simulink model "OS4dynamics_01"  (R2017b)
settings: Solver=ode45  StartTime=0.0  StopTime=10  RelTol=1e-3  EnableMultiTasking=on
InitFcn:
  | OS4dynamics_01_init
undefined symbols (not defined in the file or in its folder): Newton, OS4_initC, OS4_initR, OS4_initX, OS4_physical, Raphson
libraries: QuaternionLib x12, simulink x2
settings Model: Creator=EwingKang  LastModifiedBy=KingBoy
settings SolverCC: ZeroCrossAlgorithm=Adaptive
settings DataIOCC: LimitDataPoints=on  SaveFormat=Array  SaveOutput=off  SaveTime=off
settings OptimizationCC: DefaultParameterBehavior=Inlined  LifeSpan=inf
settings DebuggingCC: SolverPrmCheckMsg=warning  StateNameClashWarn=warning  StrictBusMsg=ErrorOnBusTreatedAsVector  SFUnexpectedBacktrackingDiag=warning  SFNoUnconditionalDefaultTransitionDiag=warning  SFExecutionAtInitializationDiag=none
settings HardwareCC: ProdBitPerPointer=32  ProdBitPerSizeT=32  ProdBitPerPtrDiffT=32  ProdLargestAtomicFloat=None  ProdIntDivRoundTo=Undefined  ProdEndianess=Unspecified  ProdWordSize=32  ProdHWDeviceType=32-bit Generic
settings ModelReferenceCC: ModelReferenceNumInstancesAllowed=Single  ModelReferencePassRootInputsByReference=off  PropagateSignalLabelsOutOfModel=off
settings CodeAppCC: StateflowObjectComments=on
settings GRTTargetCC: TargetLangStandard=C89/C90 (ANSI)  GeneratePreprocessorConditionals=Disable all
settings ConfigComp: CovMetricSettings=dw  CovHtmlReporting=on  CovSaveCumulativeToWorkspaceVar=on  CovSaveSingleToWorkspaceVar=on  CovExternalEMLEnable=off  CovSFcnEnable=off
settings SimscapeCC: EditingMode=Restricted  SimscapeNormalizeSystem=off
settings ConfigurationSet: Description=SimMechanics 2G

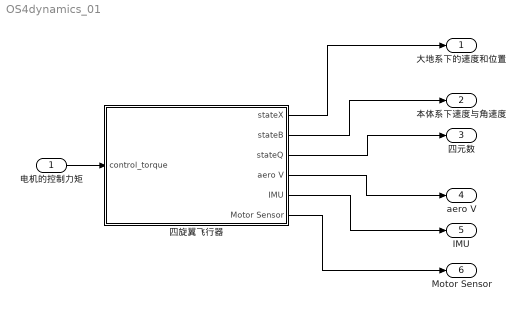
== system OS4dynamics_01 ==
  电机的控制力矩 : Inport  PortDimensions=4
  四旋翼飞行器 : Subsystem
  大地系下的速度和位置 : Outport
  本体系下速度与角速度 : Outport  Port=2
  四元数 : Outport  Port=3
  aero V : Outport  Port=4
  IMU : Outport  Port=5
  Motor Sensor : Outport  Port=6
  wires:
  电机的控制力矩/1 -> 四旋翼飞行器/1(control_torque)
  四旋翼飞行器/1(stateX) -> 大地系下的速度和位置/1
  四旋翼飞行器/2(stateB) -> 本体系下速度与角速度/1
  四旋翼飞行器/3(stateQ) -> 四元数/1
  四旋翼飞行器/4(aero V) -> aero V/1
  四旋翼飞行器/5(IMU) -> IMU/1
  四旋翼飞行器/6(Motor Sensor) -> Motor Sensor/1

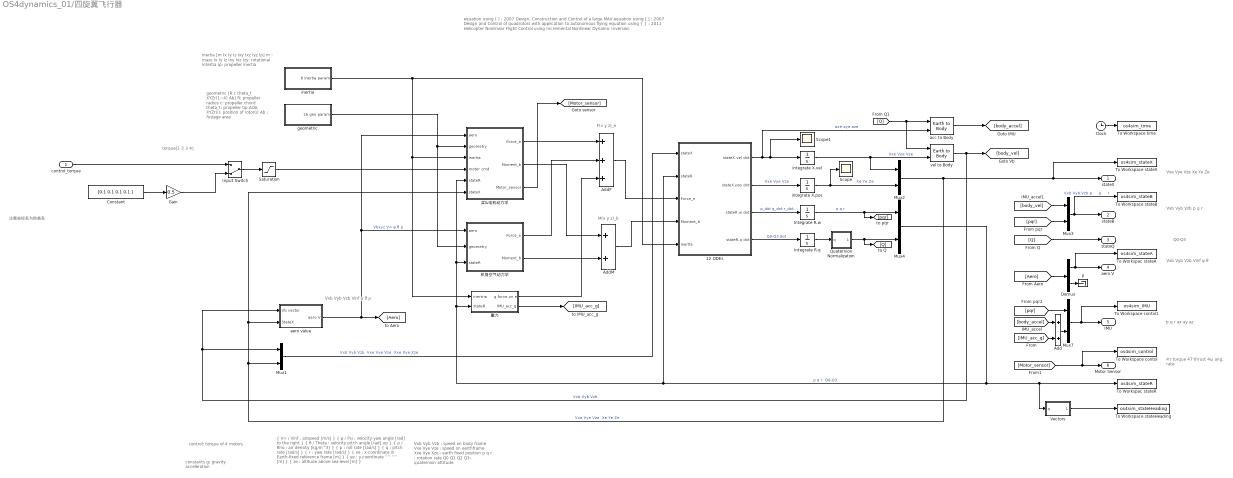
== system OS4dynamics_01/四旋翼飞行器 ==
  note: 注意坐标系为欧美系
  note: equation using ( ) : 2007 Design, Construction and Control of a large MAV
      | equation using [ ] : 2007 Design and Control of quadrotors with application to autonomous flying
      | equation using { } : 2011 Helicopter Nonlinear Flight Control using Incremental Nonlinear Dynamic Inversion
  note: Q0-Q3
  note: constants
      | g: gravity acceleration
  note: control:
      |   torque of 4 motors
  note: Vxb  Vyb Vzb : speed on body frame
      | Vxe Vye Vze  : speed on earthframe
      | Xxe Xye Xze  : earth fixed position
      | p q r               : rotation rate
      | Q0 Q1 Q2 Q3: quaternion attitude
  note: Vxb Vyb Vzb
      | p     q     r
  note: Vxe Vye Vze
      | Xe   Ye   Ze
  note: { V∞ / Vinf : airspeed [m/s] }
      | { ψ / Psi : velocity yaw angle [rad] to the right }
      | { θ / Theta : velocity pitch angle [rad] up }
      | { ρ / Rho : air density [kg/m^3] }
      | { p : roll rate [rad/s] }
      | { q : pitch rate [rad/s] }
      | { r : yaw rate [rad/s] }
      | { xe : x-coordinate in Earth-fixed reference frame [m] }
      | { ye : y-coordinate '' '' '' '' [m] }
      | { ze : altitude above sea-level [m] }
  note: torque[1 2 3 4]
  note: M(x y z)_b
  note: F(x y z)_e
  note: p q r ax ay az
  note: inertia
      | [m Ix Iy Iz Ixy Ixz Iyz Ip]
      | m : mass
      | Ix Iy Iz Ixy Ixz Izy: rotational intertia
      | Ip: propeller inertia
  note: geometric
      |  [R c theta_t XYZr(1~4) Ab]
      |
      | R:         propeller radius
      | c:          propeller chord
      | theta_t: propeller tip AOA
      | XYZr(i): position of rotor(i)
      | Ab      : fuslage area
  note: Vxb Vyb Vzb
      | Vinf ψ θ ρ
  note: Vxb Vyb Vzb
      | Vinf ψ θ
  note: 4τ torque
      | 4T thrust
      | 4ω ang. rate
  control_torque : Inport  PortDimensions=4
  12 ODEs : Subsystem
  Add : Sum
  AddF : Sum  Inputs=+++
  AddM : Sum
  Clock : Clock
  Constant : Constant  Value=[0.1 0.1 0.1 0.1 ]
  Demux : Demux  Outputs=[6 1 ]
  Gain : Gain  Gain=0.5
  Input Switch : ManualSwitch  CurrentSetting=0
  Integrate R.q : Integrator  InitialCondition=OS4_initR.q
  Integrate R.w : Integrator  InitialCondition=OS4_initR.w
  Mux{1..4,7} (5 alike) : Mux  Inputs=2
  Quaternion Normalization : Subsystem
  Saturation : Saturate  UpperLimit=0.2  LowerLimit=0
  Scope : Scope
  Scope1 : Scope
  To Workspac stateA : ToWorkspace  VariableName=os4sim_stateA  SaveFormat=Timeseries  SampleTime=-1
  To Workspac stateR : ToWorkspace  VariableName=os4sim_stateR  SaveFormat=Timeseries  SampleTime=-1
  To Workspace contol : ToWorkspace  VariableName=os4sim_control  SaveFormat=Timeseries  SampleTime=-1
  To Workspace contol1 : ToWorkspace  VariableName=os4sim_IMU  SaveFormat=Timeseries  SampleTime=-1
  To Workspace stateB : ToWorkspace  VariableName=os4sim_stateB  SaveFormat=Timeseries  SampleTime=-1
  To Workspace stateHeading : ToWorkspace  VariableName=os4sim_stateHeading  SaveFormat=Timeseries  SampleTime=-1
  To Workspace stateX : ToWorkspace  VariableName=os4sim_stateX  SaveFormat=Timeseries  SampleTime=-1
  To Workspace time : ToWorkspace  VariableName=os4sim_time  SaveFormat=Timeseries  SampleTime=-1
  Vectors : Subsystem
  acc to Body : QuaternionLib/Earth to Body
  aero value : Subsystem
  geometric : Subsystem
  inertia : Subsystem
  integrate X.pos : Integrator  InitialCondition=OS4_initX.pos
  integrate X.vel : Integrator  InitialCondition=OS4_initX.vel
  vel to Body : QuaternionLib/Earth to Body
  ρ : Terminator
  机身空气动力学 : Subsystem
  桨&电机动力学 : Subsystem
  重力 : Subsystem
  stateX : Outport
  stateB : Outport  Port=2
  stateQ : Outport  Port=3
  aero V : Outport  Port=4
  IMU : Outport  Port=5
  Motor Sensor : Outport  Port=6
  wires:
  Mux2/1 -> stateX/1, To Workspace stateX/1, 桨&电机动力学/6(stateX), aero value/2(StateX), Mux1/2  "Vxe Vye Vze  Xe Ye Ze"
  Mux1/1 -> 12 ODEs/1(stateX)  "Vxb Vyb Vzb  Vxe Vye Vze  Xxe Xye Xze"
  桨&电机动力学/1(Force_e) -> AddF/1
  Mux4/1 -> Vectors/1(q), To Workspac stateR/1, 12 ODEs/2(stateR), 重力/2(stateR), 桨&电机动力学/5(stateR), 机身空气动力学/3(stateR)  "p q r  Q0-Q3"
  12 ODEs/1(stateX.vel dot) -> acc to Body/2, Scope1/1, integrate X.vel/1  "axe aye aze"
  12 ODEs/3("stateR.w dot ") -> Integrate R.w/1  "p_dot q_dot r_dot"
  geometric/1(16 geo param) -> 机身空气动力学/2(geometry), 桨&电机动力学/2(geometry)
  aero value/1(aero V) -> [Aero], 桨&电机动力学/1(aero), 机身空气动力学/1(aero)  "Vbxyz V∞ ψ θ ρ"
  AddF/1 -> 12 ODEs/3(Force_e)
  重力/1(g force on e) -> AddF/3
  Clock/1 -> To Workspace time/1
  Quaternion Normalization/1(qnorm) -> Mux4/2, [Q]
  integrate X.vel/1 -> vel to Body/2, Mux2/1  "Vxe Vye Vze"
  vel to Body/1 -> [body_vel], aero value/1(Vb vector), Mux1/1  "Vxb Vyb Vzb"
  AddM/1 -> 12 ODEs/4(Moment_b)
  [body_accel] -> Add/1
  [Q] -> vel to Body/1, acc to Body/1
  Saturation/1 -> 桨&电机动力学/4(motor cmd)
  12 ODEs/4(stateR.q dot) -> Integrate R.q/1  "Q0-Q3 dot"
  Mux3/1 -> stateB/1, To Workspace stateB/1  "Vxb Vyb Vzb p     q     r"
  桨&电机动力学/2(Moment_b) -> AddM/1
  [Aero] -> Demux/1
  [Motor_sensor] -> Motor Sensor/1, To Workspace contol/1
  Demux/2 -> ρ/1
  control_torque/1 -> Input Switch/1
  [body_vel] -> Mux3/1
  桨&电机动力学/3(Motor_sensor) -> [Motor_sensor]
  12 ODEs/2(stateX.pos dot) -> integrate X.pos/1  "Vxe Vye Vze"
  重力/2(IMU_acc_g) -> [IMU_acc_g]
  Mux7/1 -> IMU/1, To Workspace contol1/1
  Demux/1 -> aero V/1, To Workspac stateA/1
  Integrate R.q/1 -> Quaternion Normalization/1(q)
  机身空气动力学/1(Force_e) -> AddF/2
  Add/1 -> Mux7/2
  integrate X.pos/1 -> Scope/1, Mux2/2  "Xe Ye Ze"
  Vectors/1(Vector) -> To Workspace stateHeading/1
  [Q] -> stateQ/1
  [pqr] -> Mux7/1
  [IMU_acc_g] -> Add/2
  机身空气动力学/2(Moment_b) -> AddM/2
  Integrate R.w/1 -> Mux4/1, [pqr]  "p q r"
  acc to Body/1 -> [body_accel]
  [pqr] -> Mux3/2
  Input Switch/1 -> Saturation/1
  inertia/1(8 inertia param) -> 12 ODEs/5(Inertia), 桨&电机动力学/3(inertia), 重力/1(inertria)
  Constant/1 -> Gain/1
  Gain/1 -> Input Switch/2

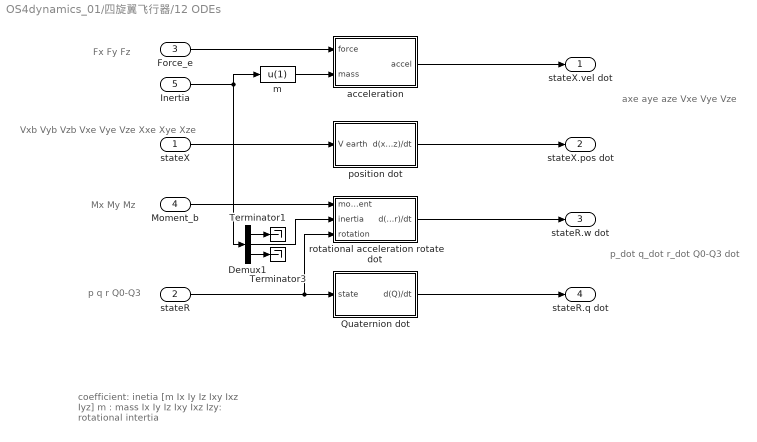
== system OS4dynamics_01/四旋翼飞行器/12 ODEs ==
  note: p_dot q_dot r_dot
      | Q0-Q3 dot
  note: axe aye aze
      | Vxe Vye Vze
  note: Vxb Vyb Vzb Vxe Vye Vze Xxe Xye Xze
  note: Mx My Mz
  note: Fx Fy Fz
  note: p q r Q0-Q3
  note: coefficient: inetia
      | [m Ix Iy Iz Ixy Ixz Iyz]
      | m : mass
      | Ix Iy Iz Ixy Ixz Izy: rotational intertia
  stateX : Inport
  stateR : Inport  Port=2
  Force_e : Inport  Port=3
  Moment_b : Inport  Port=4
  Inertia : Inport  Port=5
  Demux1 : Demux  Outputs=[1 3 4]
  Quaternion dot : Subsystem
  Terminator1 : Terminator
  Terminator3 : Terminator
  acceleration : Subsystem
  m : Fcn  Expr=u(1)
  position dot : Subsystem
  rotational acceleration rotate dot : Subsystem
  stateX.vel dot : Outport
  stateX.pos dot : Outport  Port=2
  "stateR.w dot " : Outport  Port=3
  stateR.q dot : Outport  Port=4
  wires:
  Inertia/1 -> m/1, Demux1/1
  Moment_b/1 -> rotational acceleration rotate dot/1(moment)
  Force_e/1 -> acceleration/1(force)
  stateR/1 -> rotational acceleration rotate dot/3(rotation), Quaternion dot/1(state)
  acceleration/1(accel) -> stateX.vel dot/1
  position dot/1(d(xyz)/dt) -> stateX.pos dot/1
  rotational acceleration rotate dot/1(d(pqr)/dt) -> "stateR.w dot "/1
  stateX/1 -> position dot/1(V earth)
  m/1 -> acceleration/2(mass)
  Demux1/2 -> rotational acceleration rotate dot/2(inertia)
  Demux1/1 -> Terminator1/1
  Demux1/3 -> Terminator3/1
  Quaternion dot/1(d(Q)/dt) -> stateR.q dot/1

== system OS4dynamics_01/四旋翼飞行器/Quaternion Normalization ==
  q : Inport  PortDimensions=4
  Product : Product  Inputs=*/  SaturateOnIntegerOverflow=on  RndMeth=Zero  InputSameDT=on  OutDataTypeStr=Inherit: Same as first input
  Square : Math  Operator=square  SaturateOnIntegerOverflow=on
  Square Root : Sqrt  Operator=signedSqrt  AlgorithmType=Newton-Raphson  SaturateOnIntegerOverflow=on
  Sum : Sum  Inputs=1  SaturateOnIntegerOverflow=on  InputSameDT=on  OutDataTypeStr=Inherit: Same as first input
  qnorm : Outport  PortDimensions=4
  wires:
  Product/1 -> qnorm/1
  Square Root/1 -> Product/2
  Square/1 -> Sum/1
  Sum/1 -> Square Root/1
  q/1 -> Product/1, Square/1

== system OS4dynamics_01/四旋翼飞行器/Vectors ==
  q : Inport
  1,0,0 : Subsystem
  1,0,1 : Subsystem
  Body to Earth w/R1 : QuaternionLib/Body to Earth w//R
  Body to Earth w/R2 : QuaternionLib/Body to Earth w//R
  Mux6 : Mux  Inputs=2
  Vector : Outport
  wires:
  1,0,0/1(1,0,0) -> Body to Earth w/R1/2
  Body to Earth w/R1/1 -> Mux6/1
  q/1 -> Body to Earth w/R1/1, Body to Earth w/R2/1  "p q r  Q0-Q3"
  Mux6/1 -> Vector/1
  Body to Earth w/R2/1 -> Mux6/2
  1,0,1/1(0,1,0) -> Body to Earth w/R2/2

== system OS4dynamics_01/四旋翼飞行器/aero value ==
  note: Vxb Vyb Vzb
      | Vinf
      | ψ
      | θ
      | ρ
  note: Vxb Vyb Vzb
  Vb vector : Inport
  StateX : Inport  Port=2
  Compare To Constant : simulink/Logic and Bit Operations/Compare To Constant  relop=>  const=0  OutDataTypeStr=boolean
  Constant : Constant  Value=inf
  Mux : Mux  Inputs=5
  Mux1 : Mux  Inputs=2
  Switch : Switch  Criteria=u2 > Threshold
  Vinf alpha beta : Display
  Vinfinity : Fcn  Expr=sqrt(u(1)^2+u(2)^2+u(3)^2)
  Vx Vy Vz : Display
  altitude air density : Fcn  Expr=1.23
  θ asin ( -Vz / Vinf) : Fcn  Expr=asin(-u(4) / u(1))
  ψ atan( Vy / Vx ) : Fcn  Expr=atan2( u(2),u(1) )
  aero V : Outport
  wires:
  Switch/1 -> Mux/2, Mux1/1
  θ asin ( -Vz / Vinf)/1 -> Mux/4
  Mux/1 -> Vinf alpha beta/1, aero V/1
  ψ atan( Vy / Vx )/1 -> Mux/3
  Mux1/1 -> θ asin ( -Vz / Vinf)/1
  altitude air density/1 -> Mux/5
  StateX/1 -> altitude air density/1
  Vb vector/1 -> Vinfinity/1, ψ atan( Vy / Vx )/1, Mux1/2, Vx Vy Vz/1, Mux/1
  Vinfinity/1 -> Switch/1, Compare To Constant/1
  Compare To Constant/1 -> Switch/2
  Constant/1 -> Switch/3

== system OS4dynamics_01/四旋翼飞行器/geometric ==
  note: geometric
      |  [R c theta_t XYZr(1~4) Ab]
      |
      | R:         propeller radius
      | c:          propeller chord
      | theta_t: propeller tip AOA
      | XYZr(i): position of rotor(i)
      | Ab      : fuslage area
  Mux6 : Mux  Inputs=8
  Propeller Chord c : Constant  Value=OS4_physical.prop.chord
  Propeller tip AOA : Constant  Value=OS4_physical.prop.thetatip
  body area Ab : Constant  Value=OS4_physical.size.fuselage.area
  propeller Radius R : Constant  Value=OS4_physical.prop.rad
  rotor1 pos XYZr1 : Constant  Value=OS4_physical.rotor.pos(1:3,1)
  rotor1 pos XYZr2 : Constant  Value=OS4_physical.rotor.pos(1:3,2)
  rotor1 pos XYZr3 : Constant  Value=OS4_physical.rotor.pos(1:3,3)
  rotor1 pos XYZr4 : Constant  Value=OS4_physical.rotor.pos(1:3,4)
  16 geo param : Outport
  wires:
  Mux6/1 -> 16 geo param/1
  propeller Radius R/1 -> Mux6/1
  Propeller Chord c/1 -> Mux6/3
  rotor1 pos XYZr1/1 -> Mux6/4
  rotor1 pos XYZr2/1 -> Mux6/5
  rotor1 pos XYZr3/1 -> Mux6/6
  rotor1 pos XYZr4/1 -> Mux6/7
  body area Ab/1 -> Mux6/8
  Propeller tip AOA/1 -> Mux6/2

== system OS4dynamics_01/四旋翼飞行器/inertia ==
  note: inertia
      | [m Ix Iy Iz Ixy Ixz Iyz Ip]
      | m : mass
      | Ix Iy Iz Ixy Ixz Izy: rotational intertia
      | Ip: propeller inertia
  Ip : Constant  Value=OS4_physical.inertia.Ip
  Ix : Constant  Value=OS4_physical.inertia.Ixx
  Ixy : Constant  Value=OS4_physical.inertia.Ixy
  Ixz : Constant  Value=OS4_physical.inertia.Ixz
  Iy : Constant  Value=OS4_physical.inertia.Iyy
  Iyz : Constant  Value=OS4_physical.inertia.Iyz
  Iz : Constant  Value=OS4_physical.inertia.Izz
  Mux : Mux  Inputs=2
  Mux1 : Mux  Inputs=2
  Mux2 : Mux  Inputs=2
  Mux6 : Mux  Inputs=5
  m : Constant  Value=OS4_physical.inertia.mass
  8 inertia param : Outport
  wires:
  Ix/1 -> Mux/1
  Iy/1 -> Mux/2
  Ixz/1 -> Mux2/1
  Iyz/1 -> Mux2/2
  Iz/1 -> Mux1/1
  Ixy/1 -> Mux1/2
  Mux6/1 -> 8 inertia param/1
  m/1 -> Mux6/1
  Mux/1 -> Mux6/2
  Mux1/1 -> Mux6/3
  Mux2/1 -> Mux6/4
  Ip/1 -> Mux6/5

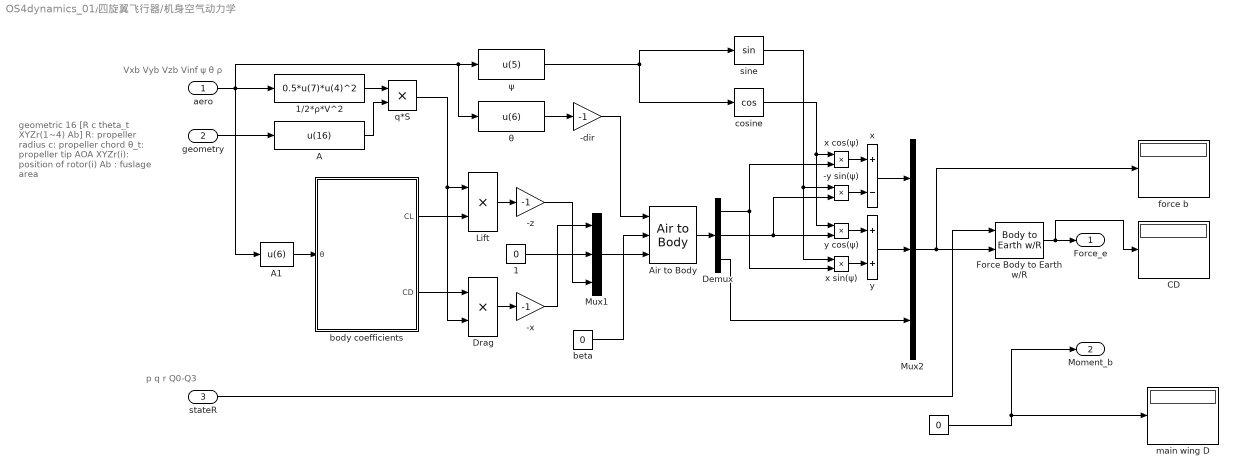
== system OS4dynamics_01/四旋翼飞行器/机身空气动力学 ==
  note: p q r
      | Q0-Q3
  note: Vxb Vyb Vzb
      | Vinf ψ θ ρ
  note: geometric 16
      | [R c theta_t XYZr(1~4) Ab]
      |
      | R: propeller radius
      | c: propeller chord
      | θ_t: propeller tip AOA
      | XYZr(i): position of rotor(i)
      | Ab : fuslage area
  aero : Inport  PortDimensions=7
  geometry : Inport  Port=2
  stateR : Inport  Port=3
  "  " : Constant  Value=0
  " 1" : Constant  Value=0
  -dir : Gain  Gain=-1
  -x : Gain  Gain=-1
  -y sin(ψ) : Product
  -z : Gain  Gain=-1
  1/2*ρ*V^2 : Fcn  Expr=0.5*u(7)*u(4)^2
  A : Fcn  Expr=u(16)
  A1 : Fcn  Expr=u(6)
  Air to Body : QuaternionLib/Air to Body
  CD : Display
  Demux : Demux  Outputs=3
  Drag : Product
  Force Body to Earth w/R : QuaternionLib/Body to Earth w//R
  Lift : Product
  Mux1 : Mux  Inputs=3
  Mux2 : Mux  Inputs=3
  beta : Constant  Value=0
  body coefficients : Subsystem
  cosine : Trigonometry  Operator=cos
  force b : Display
  main wing D : Display
  q*S : Product
  sine : Trigonometry
  x : Sum  Inputs=+-
  x cos(ψ) : Product
  x sin(ψ) : Product
  y : Sum
  y cos(ψ) : Product
  θ : Fcn  Expr=u(6)
  ψ : Fcn  Expr=u(5)
  Force_e : Outport
  Moment_b : Outport  Port=2
  wires:
  Force Body to Earth w/R/1 -> CD/1, Force_e/1
  stateR/1 -> Force Body to Earth w/R/1
  geometry/1 -> A/1
  1/2*ρ*V^2/1 -> q*S/1
  A/1 -> q*S/2
  q*S/1 -> Lift/1, Drag/2
  "  "/1 -> main wing D/1, Moment_b/1
  aero/1 -> A1/1, θ/1, ψ/1, 1/2*ρ*V^2/1
  body coefficients/2(CD) -> Drag/1
  body coefficients/1(CL) -> Lift/2
  A1/1 -> body coefficients/1(θ)
  Drag/1 -> -x/1
  -x/1 -> Mux1/1
  Lift/1 -> -z/1
  -z/1 -> Mux1/3
  " 1"/1 -> Mux1/2
  θ/1 -> -dir/1
  -dir/1 -> Air to Body/1
  Mux1/1 -> Air to Body/3
  beta/1 -> Air to Body/2
  Air to Body/1 -> Demux/1
  ψ/1 -> sine/1, cosine/1
  x/1 -> Mux2/1
  y/1 -> Mux2/2
  cosine/1 -> y cos(ψ)/1, x cos(ψ)/1
  Demux/1 -> x sin(ψ)/2, x cos(ψ)/2
  Demux/3 -> Mux2/3
  x sin(ψ)/1 -> y/2
  x cos(ψ)/1 -> x/1
  -y sin(ψ)/1 -> x/2
  y cos(ψ)/1 -> y/1
  Demux/2 -> -y sin(ψ)/2, y cos(ψ)/2
  sine/1 -> -y sin(ψ)/1, x sin(ψ)/1
  Mux2/1 -> force b/1, Force Body to Earth w/R/2

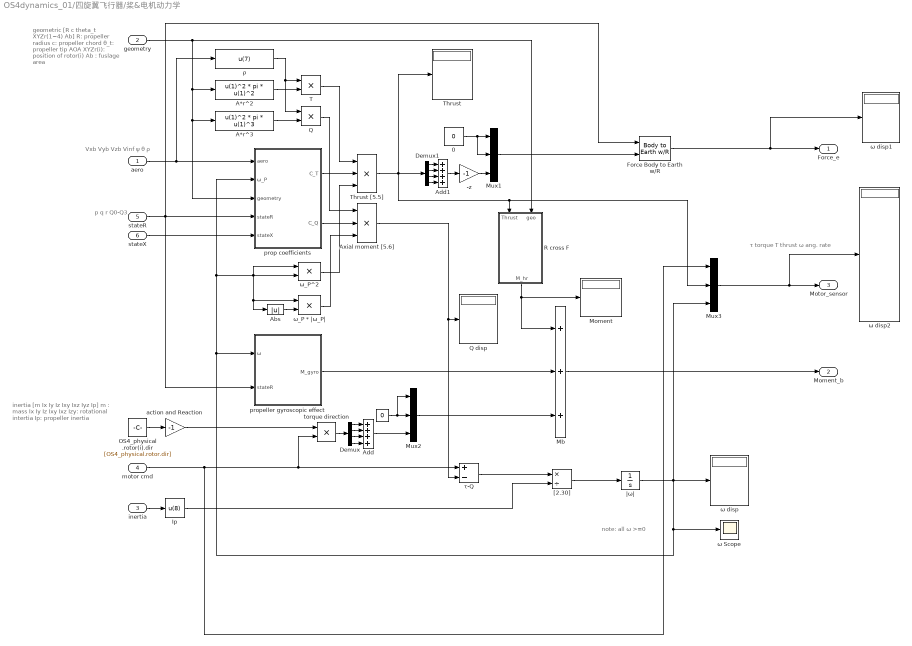
== system OS4dynamics_01/四旋翼飞行器/桨&电机动力学 ==
  note: τ torque
      | T thrust
      | ω ang. rate
  note: note: all ω >=0
  note: p q r
      | Q0-Q3
  note: Vxb Vyb Vzb
      | Vinf ψ θ ρ
  note: geometric
      | [R c theta_t XYZr(1~4) Ab]
      |
      | R: propeller radius
      | c: propeller chord
      | θ_t: propeller tip AOA
      | XYZr(i): position of rotor(i)
      | Ab : fuslage area
  note: inertia
      | [m Ix Iy Iz Ixy Ixz Iyz Ip]
      | m : mass
      | Ix Iy Iz Ixy Ixz Izy: rotational intertia
      | Ip: propeller inertia
  aero : Inport  PortDimensions=7
  geometry : Inport  Port=2
  inertia : Inport  Port=3
  motor cmd : Inport  Port=4
  stateR : Inport  Port=5  PortDimensions=7
  stateX : Inport  Port=6  PortDimensions=6
  "  " : Constant  Value=0
  " τ-Q" : Sum  Inputs=+-
  -z : Gain  Gain=-1
  0 : Constant  Value=0
  A*r^2 : Fcn  Expr=u(1)^2 * pi * u(1)^2
  A*r^3 : Fcn  Expr=u(1)^2 * pi * u(1)^3
  Abs : Abs
  Add : Sum  Inputs=++++
  Add1 : Sum  Inputs=++++
  Axial moment [5.6] : Product  Inputs=3
  Demux : Demux
  Demux1 : Demux
  Force Body to Earth w/R : QuaternionLib/Body to Earth w//R
  Ip : Fcn  Expr=u(8)
  Mb : Sum  Inputs=+++
  Moment : Display
  Mux1 : Mux  Inputs=3
  Mux2 : Mux  Inputs=3
  Mux3 : Mux  Inputs=3
  OS4_physical .rotor(i).dir : Constant  Value=[OS4_physical.rotor.dir]
  Q : Product
  Q disp : Display
  R cross F : MATLAB Function  TreatAsAtomicUnit=on
  T : Product
  Thrust : Display
  Thrust [5.5] : Product  Inputs=3
  "[2.30]" : Product  Inputs=*/
  action and Reaction : Gain  Gain=-1
  prop coefficients : Subsystem
  propeller gyroscopic effect : Subsystem
  torque direction : Product
  |ω| : Integrator  InitialCondition=OS4_initC.rotor.omega
  ρ : Fcn  Expr=u(7)
  ω Scope : Scope
  ω disp : Display
  ω disp1 : Display
  ω disp2 : Display
  ω_P * |ω_P| : Product
  ω_P^2 : Product
  Force_e : Outport
  Moment_b : Outport  Port=2
  Motor_sensor : Outport  Port=3
  wires:
  Force Body to Earth w/R/1 -> ω disp1/1, Force_e/1
  stateR/1 -> Force Body to Earth w/R/1, propeller gyroscopic effect/2(stateR), prop coefficients/4(stateR)
  geometry/1 -> R cross F/2(geo), prop coefficients/3(geometry), A*r^3/1, A*r^2/1
  ρ/1 -> Q/1, T/1
  A*r^2/1 -> T/2
  T/1 -> Thrust [5.5]/1
  Mb/1 -> Moment_b/1
  aero/1 -> prop coefficients/1(aero), ρ/1
  prop coefficients/1(C_T) -> Thrust [5.5]/2
  ω_P^2/1 -> Thrust [5.5]/3
  A*r^3/1 -> Q/2
  Q/1 -> Axial moment [5.6]/1
  Abs/1 -> ω_P * |ω_P|/2
  prop coefficients/2(C_Q) -> Axial moment [5.6]/2
  ω_P * |ω_P|/1 -> Axial moment [5.6]/3
  -z/1 -> Mux1/3
  0/1 -> Mux1/1, Mux1/2
  OS4_physical .rotor(i).dir/1 -> action and Reaction/1
  action and Reaction/1 -> torque direction/1
  Axial moment [5.6]/1 -> Q disp/1, " τ-Q"/2
  motor cmd/1 -> Mux3/1, " τ-Q"/1, torque direction/2
  " τ-Q"/1 -> "[2.30]"/1
  inertia/1 -> Ip/1
  Ip/1 -> "[2.30]"/2
  "[2.30]"/1 -> |ω|/1
  torque direction/1 -> Demux/1
  Mux2/1 -> Mb/3
  propeller gyroscopic effect/1(M_gyro) -> Mb/2
  "  "/1 -> Mux2/1, Mux2/2
  R cross F/1(M_hr) -> Mb/1, Moment/1
  Mux1/1 -> Force Body to Earth w/R/2
  stateX/1 -> prop coefficients/5(stateX)
  Demux/1 -> Add/1
  Demux/2 -> Add/2
  Demux/3 -> Add/3
  Demux/4 -> Add/4
  Add/1 -> Mux2/3
  Thrust [5.5]/1 -> Mux3/2, R cross F/1(Thrust), Thrust/1, Demux1/1
  Demux1/1 -> Add1/1
  Demux1/2 -> Add1/2
  Demux1/3 -> Add1/3
  Demux1/4 -> Add1/4
  Add1/1 -> -z/1
  |ω|/1 -> propeller gyroscopic effect/1(ω), Abs/1, ω_P * |ω_P|/1, ω_P^2/2, ω_P^2/1, prop coefficients/2(ω_P), ω Scope/1, Mux3/3, ω disp/1
  Mux3/1 -> ω disp2/1, Motor_sensor/1

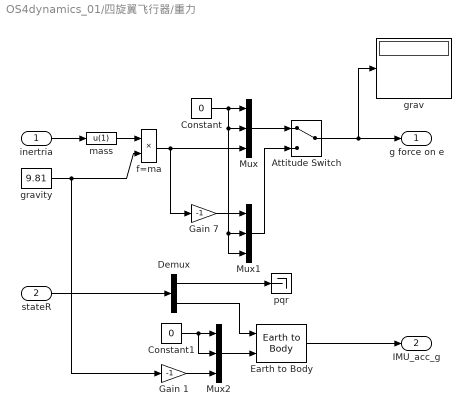
== system OS4dynamics_01/四旋翼飞行器/重力 ==
  inertria : Inport
  stateR : Inport  Port=2
  " mass" : Fcn  Expr=u(1)
  Attitude Switch : ManualSwitch
  Constant : Constant  Value=0
  Constant1 : Constant  Value=0
  Demux : Demux  Outputs=[3 4]
  Earth to Body : QuaternionLib/Earth to Body
  Gain 1 : Gain  Gain=-1  SaturateOnIntegerOverflow=on  OutDataTypeStr=Inherit: Same as input  ParamDataTypeStr=Inherit: Same as input
  Gain 7 : Gain  Gain=-1  SaturateOnIntegerOverflow=on  OutDataTypeStr=Inherit: Same as input  ParamDataTypeStr=Inherit: Same as input
  Mux : Mux  Inputs=3
  Mux1 : Mux  Inputs=3
  Mux2 : Mux  Inputs=3
  f=ma : Product  Inputs=**
  grav : Display
  gravity : Constant  Value=9.81
  pqr : Terminator
  g force on e : Outport
  IMU_acc_g : Outport  Port=2
  wires:
  Attitude Switch/1 -> g force on e/1, grav/1
  " mass"/1 -> f=ma/1
  Constant/1 -> Mux/1, Mux1/3, Mux1/2, Mux/2
  inertria/1 -> " mass"/1
  Mux/1 -> Attitude Switch/1
  Mux1/1 -> Attitude Switch/2
  Gain 7/1 -> Mux1/1
  Earth to Body/1 -> IMU_acc_g/1
  Constant1/1 -> Mux2/1, Mux2/2
  Mux2/1 -> Earth to Body/2
  stateR/1 -> Demux/1
  Demux/2 -> Earth to Body/1
  Demux/1 -> pqr/1
  Gain 1/1 -> Mux2/3
  gravity/1 -> f=ma/2, Gain 1/1
  f=ma/1 -> Mux/3, Gain 7/1

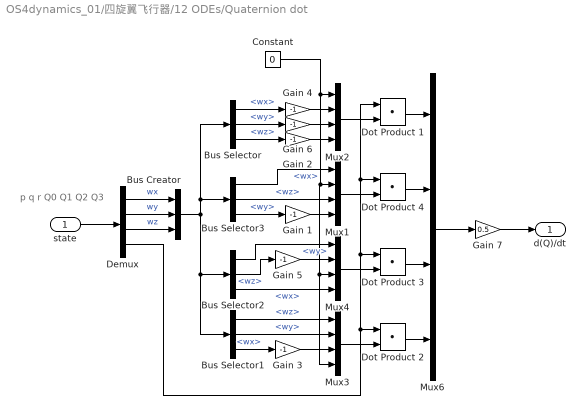
== system OS4dynamics_01/四旋翼飞行器/12 ODEs/Quaternion dot ==
  note: p q r Q0 Q1 Q2 Q3
  state : Inport
  Bus Creator : BusCreator  Inputs=3
  Bus Selector : BusSelector  OutputSignals=wx,wy,wz
  Bus Selector1 : BusSelector  OutputSignals=wz,wy,wx
  Bus Selector2 : BusSelector  OutputSignals=wy,wz,wx
  Bus Selector3 : BusSelector  OutputSignals=wx,wz,wy
  Constant : Constant  Value=0
  Demux : Demux  Outputs=[1 1 1 4]
  Dot Product {1..4} (4 alike) : DotProduct  InputSameDT=on  OutDataTypeStr=Inherit: Inherit via internal rule
  Gain {1..6} (6 alike) : Gain  Gain=-1  SaturateOnIntegerOverflow=on  OutDataTypeStr=Inherit: Same as input  ParamDataTypeStr=Inherit: Same as input
  Gain 7 : Gain  Gain=0.5  SaturateOnIntegerOverflow=on  OutDataTypeStr=Inherit: Same as input  ParamDataTypeStr=Inherit: Same as input
  Mux{1..4,6} (5 alike) : Mux
  d(Q)/dt : Outport
  wires:
  Mux6/1 -> Gain 7/1
  state/1 -> Demux/1
  Gain 2/1 -> Mux2/4
  Bus Selector/1 -> Gain 4/1  "<wx>"
  Mux2/1 -> Dot Product 1/2
  Mux3/1 -> Dot Product 2/2
  Mux4/1 -> Dot Product 3/2
  Demux/1 -> Bus Creator/1  "wx"
  Demux/2 -> Bus Creator/2  "wy"
  Demux/3 -> Bus Creator/3  "wz"
  Gain 5/1 -> Mux4/2
  Gain 3/1 -> Mux3/3
  Mux1/1 -> Dot Product 4/2
  Bus Creator/1 -> Bus Selector2/1, Bus Selector1/1, Bus Selector/1, Bus Selector3/1
  Constant/1 -> Mux2/1, Mux1/2, Mux3/4, Mux4/3
  Bus Selector3/3 -> Gain 1/1  "<wy>"
  Gain 4/1 -> Mux2/2
  Gain 6/1 -> Mux2/3
  Bus Selector/2 -> Gain 6/1  "<wy>"
  Bus Selector/3 -> Gain 2/1  "<wz>"
  Dot Product 2/1 -> Mux6/4
  Dot Product 3/1 -> Mux6/3
  Dot Product 4/1 -> Mux6/2
  Dot Product 1/1 -> Mux6/1
  Demux/4 -> Dot Product 3/1, Dot Product 4/1, Dot Product 1/1, Dot Product 2/1
  Gain 7/1 -> d(Q)/dt/1
  Bus Selector3/1 -> Mux1/1  "<wx>"
  Bus Selector3/2 -> Mux1/3  "<wz>"
  Gain 1/1 -> Mux1/4
  Bus Selector1/3 -> Gain 3/1  "<wx>"
  Bus Selector1/2 -> Mux3/2  "<wy>"
  Bus Selector1/1 -> Mux3/1  "<wz>"
  Bus Selector2/1 -> Mux4/1  "<wy>"
  Bus Selector2/2 -> Gain 5/1  "<wz>"
  Bus Selector2/3 -> Mux4/4  "<wx>"

== system OS4dynamics_01/四旋翼飞行器/12 ODEs/acceleration ==
  force : Inport
  mass : Inport  Port=2
  Mux : Mux  Inputs=2
  Mux1 : Mux  Inputs=3
  x : Fcn  Expr=u(1)/u(4)
  y : Fcn  Expr=u(2)/u(4)
  z : Fcn  Expr=u(3)/u(4)
  accel : Outport
  wires:
  force/1 -> Mux/1
  Mux/1 -> z/1, y/1, x/1
  Mux1/1 -> accel/1
  x/1 -> Mux1/1
  y/1 -> Mux1/2
  z/1 -> Mux1/3
  mass/1 -> Mux/2

== system OS4dynamics_01/四旋翼飞行器/12 ODEs/position dot ==
  V earth : Inport
  Demux : Demux  Outputs=[3 3 3]
  Mux1 : Mux  Inputs=3
  Terminator1 : Terminator
  Terminator2 : Terminator
  Vx : Fcn  Expr=u(1)
  Vy : Fcn  Expr=u(2)
  Vz : Fcn  Expr=u(3)
  d(xyz)/dt : Outport
  wires:
  Mux1/1 -> d(xyz)/dt/1
  V earth/1 -> Demux/1
  Demux/3 -> Terminator1/1
  Demux/1 -> Terminator2/1
  Demux/2 -> Vz/1, Vx/1, Vy/1
  Vx/1 -> Mux1/1
  Vy/1 -> Mux1/2
  Vz/1 -> Mux1/3

== system OS4dynamics_01/四旋翼飞行器/12 ODEs/rotational acceleration rotate dot ==
  note: 1 Mx My Mz
      | 4 Ix Iy Iz
      | 7p q r
  moment : Inport
  inertia : Inport  Port=2
  rotation : Inport  Port=3
  Demux1 : Demux  Outputs=[3 4]
  Mux : Mux  Inputs=3
  Mux1 : Mux  Inputs=3
  Terminator3 : Terminator
  p dot : Fcn  Expr=((u(5)-u(6))*u(8)*u(9) + u(1))/u(4)
  q dot : Fcn  Expr=((u(6)-u(4))*u(7)*u(9) + u(2)) / u(5)
  r dot : Fcn  Expr=((u(4)-u(5))*u(7)*u(8) + u(3)) / u(6)
  d(pqr)/dt : Outport
  wires:
  moment/1 -> Mux/1
  Mux/1 -> r dot/1, q dot/1, p dot/1
  Mux1/1 -> d(pqr)/dt/1
  p dot/1 -> Mux1/1
  q dot/1 -> Mux1/2
  r dot/1 -> Mux1/3
  inertia/1 -> Mux/2
  rotation/1 -> Demux1/1
  Demux1/1 -> Mux/3
  Demux1/2 -> Terminator3/1

== system OS4dynamics_01/四旋翼飞行器/Vectors/1,0,0 ==
  Ixy : Constant  Value=0
  Ixz : Constant  Value=0
  Mux6 : Mux  Inputs=3
  m : Constant
  1,0,0 : Outport
  wires:
  Mux6/1 -> 1,0,0/1
  m/1 -> Mux6/1
  Ixy/1 -> Mux6/3
  Ixz/1 -> Mux6/2

== system OS4dynamics_01/四旋翼飞行器/Vectors/1,0,1 ==
  Ixy : Constant  Value=0
  Ixz : Constant
  Mux6 : Mux  Inputs=3
  m : Constant  Value=0
  0,1,0 : Outport
  wires:
  Mux6/1 -> 0,1,0/1
  m/1 -> Mux6/1
  Ixy/1 -> Mux6/3
  Ixz/1 -> Mux6/2

== system OS4dynamics_01/四旋翼飞行器/机身空气动力学/body coefficients ==
  θ : Inport
  2θ1 : Gain  Gain=2
  Add : Sum
  Gain1 : Gain  Gain=-0.45
  cos(θ) : Trigonometry  Operator=cos
  max 0.5 min 0 : Gain  Gain=0.5
  max 0.65 min 0.2 : Constant  Value=0.45+0.2
  sin(2θ) : Trigonometry
  CL : Outport
  CD : Outport  Port=2
  wires:
  sin(2θ)/1 -> max 0.5 min 0/1
  max 0.5 min 0/1 -> CL/1
  cos(θ)/1 -> Gain1/1
  Gain1/1 -> Add/1
  θ/1 -> cos(θ)/1, 2θ1/1
  Add/1 -> CD/1
  max 0.65 min 0.2/1 -> Add/2
  2θ1/1 -> sin(2θ)/1

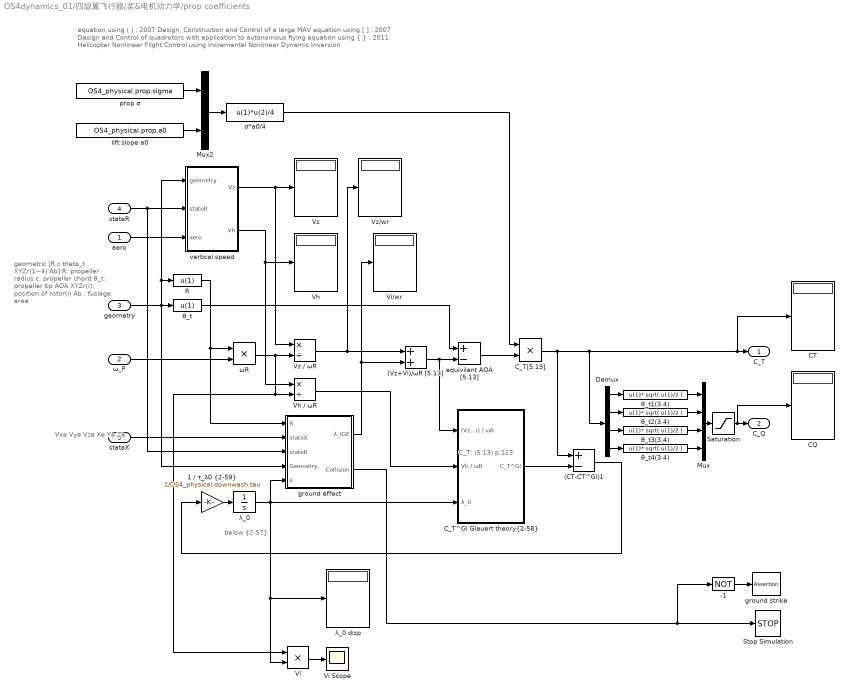
== system OS4dynamics_01/四旋翼飞行器/桨&电机动力学/prop coefficients ==
  note: Vxe Vye Vze
      |  Xe Ye Ze
  note: below {2-57}
  note: C_T: (5.13) p.123
  note: geometric
      | [R c theta_t XYZr(1~4) Ab]
      |
      | R: propeller radius
      | c: propeller chord
      | θ_t: propeller tip AOA
      | XYZr(i): position of rotor(i)
      | Ab : fuslage area
  note: equation using ( ) : 2007 Design, Construction and Control of a large MAV
      | equation using [ ] : 2007 Design and Control of quadrotors with application to autonomous flying
      | equation using { } : 2011 Helicopter Nonlinear Flight Control using Incremental Nonlinear Dynamic Inversion
  aero : Inport
  ω_P : Inport  Port=2  PortDimensions=4
  geometry : Inport  Port=3
  stateR : Inport  Port=4
  stateX : Inport  Port=5
  (CT-CT^Gl)1 : Sum  Inputs=+-
  (Vz+Vi)/ωR [5.13] : Sum
  -1 : Logic  Operator=NOT  AllPortsSameDT=off  OutDataTypeStr=boolean
  "1 / τ_λ0 {2-59}" : Gain  Gain=1/OS4_physical.downwash.tau
  CQ : Display
  CT : Display
  C_T[5.13] : Product
  "C_T^Gl Glauert theory{2-58}" : Subsystem
  Demux : Demux
  Mux : Mux
  Mux2 : Mux  Inputs=2
  R : Fcn  Expr=u(1)
  Saturation : Saturate  UpperLimit=inf  LowerLimit=0.001
  Stop Simulation : Stop
  Vh : Display
  Vh / ωR : Product  Inputs=*/
  Vi : Product  Inputs=**
  Vi Scope : Scope
  Vi/wr : Display
  Vz : Display
  Vz / ωR : Product  Inputs=*/
  Vz/wr : Display
  equivilant AOA [5.13] : Sum  Inputs=+-
  ground effect : Subsystem
  ground strike : Assertion  AssertionFailFcn=error('Ground Collision!!')  StopWhenAssertionFail=off
  lift slope a0 : Constant  Value=OS4_physical.prop.a0
  prop σ : Constant  Value=OS4_physical.prop.sigma
  vertical speed : Subsystem
  θ_t : Fcn  Expr=u(1)
  θ_t1(3.4) : Fcn  Expr=u(1)* sqrt( u(1)/2 )
  θ_t2(3.4) : Fcn  Expr=u(1)* sqrt( u(1)/2 )
  θ_t3(3.4) : Fcn  Expr=u(1)* sqrt( u(1)/2 )
  θ_t4(3.4) : Fcn  Expr=u(1)* sqrt( u(1)/2 )
  λ_0 : Integrator  InitialCondition=OS4_initC.propeller.lambda_0
  λ_0 disp : Display
  σ*a0/4 : Fcn  Expr=u(1)*u(2)/4
  ωR : Product
  C_T : Outport
  C_Q : Outport  Port=2
  wires:
  C_T[5.13]/1 -> CT/1, C_T/1, Demux/1, (CT-CT^Gl)1/1
  Saturation/1 -> CQ/1, C_Q/1
  geometry/1 -> vertical speed/1(geometry), R/1, ground effect/4(Geometry), θ_t/1
  ω_P/1 -> ωR/2
  R/1 -> ωR/1, ground effect/1(R)
  lift slope a0/1 -> Mux2/2
  prop σ/1 -> Mux2/1
  θ_t/1 -> equivilant AOA [5.13]/1
  Mux2/1 -> σ*a0/4/1
  σ*a0/4/1 -> C_T[5.13]/1
  equivilant AOA [5.13]/1 -> C_T[5.13]/2
  ωR/1 -> Vz / ωR/2, Vi/1, Vh / ωR/2
  Vz / ωR/1 -> Vz/wr/1, (Vz+Vi)/ωR [5.13]/1
  (Vz+Vi)/ωR [5.13]/1 -> "C_T^Gl Glauert theory{2-58}"/1((Vz+Vi) / ωR), equivilant AOA [5.13]/2
  stateR/1 -> vertical speed/2(stateR), ground effect/3(stateR)
  aero/1 -> vertical speed/3(aero)
  "1 / τ_λ0 {2-59}"/1 -> λ_0/1
  (CT-CT^Gl)1/1 -> "1 / τ_λ0 {2-59}"/1
  vertical speed/1(Vz) -> Vz/1, Vz / ωR/1
  vertical speed/2(Vh) -> Vh/1, Vh / ωR/1
  "C_T^Gl Glauert theory{2-58}"/1(C_T^Gl) -> (CT-CT^Gl)1/2
  Vh / ωR/1 -> "C_T^Gl Glauert theory{2-58}"/2(Vh / ωR)
  θ_t1(3.4)/1 -> Mux/1
  λ_0/1 -> Vi/2, λ_0 disp/1, ground effect/5(λ), "C_T^Gl Glauert theory{2-58}"/3(λ_0)
  stateX/1 -> ground effect/2(stateX)
  ground effect/1(λ_IGE) -> Vi/wr/1, (Vz+Vi)/ωR [5.13]/2
  ground effect/2(Collision) -> -1/1, Stop Simulation/1
  -1/1 -> ground strike/1
  Vi/1 -> Vi Scope/1
  Demux/1 -> θ_t1(3.4)/1
  Demux/2 -> θ_t2(3.4)/1
  Demux/3 -> θ_t3(3.4)/1
  Demux/4 -> θ_t4(3.4)/1
  θ_t2(3.4)/1 -> Mux/2
  Mux/1 -> Saturation/1
  θ_t3(3.4)/1 -> Mux/3
  θ_t4(3.4)/1 -> Mux/4

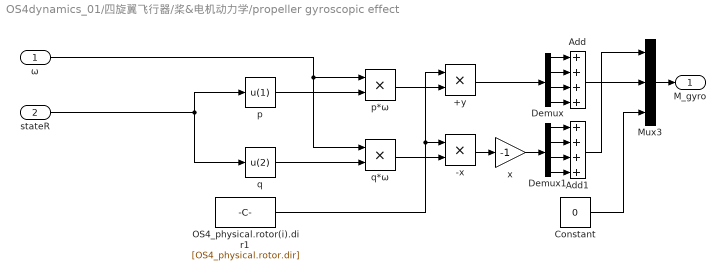
== system OS4dynamics_01/四旋翼飞行器/桨&电机动力学/propeller gyroscopic effect ==
  ω : Inport  PortDimensions=4
  stateR : Inport  Port=2
  +y : Product
  -x : Product
  Add : Sum  Inputs=++++
  Add1 : Sum  Inputs=++++
  Constant : Constant  Value=0
  Demux : Demux
  Demux1 : Demux
  Mux3 : Mux  Inputs=3
  OS4_physical.rotor(i).dir1 : Constant  Value=[OS4_physical.rotor.dir]
  p : Fcn  Expr=u(1)
  p*ω : Product
  q : Fcn  Expr=u(2)
  q*ω : Product
  x : Gain  Gain=-1
  M_gyro : Outport
  wires:
  x/1 -> Demux1/1
  q*ω/1 -> -x/2
  q/1 -> q*ω/2
  p/1 -> p*ω/2
  OS4_physical.rotor(i).dir1/1 -> +y/1, -x/1
  +y/1 -> Demux/1
  -x/1 -> x/1
  ω/1 -> q*ω/1, p*ω/1
  Mux3/1 -> M_gyro/1
  stateR/1 -> p/1, q/1
  p*ω/1 -> +y/2
  Demux/1 -> Add/1
  Demux/2 -> Add/2
  Demux/3 -> Add/3
  Demux/4 -> Add/4
  Demux1/1 -> Add1/1
  Demux1/2 -> Add1/2
  Demux1/3 -> Add1/3
  Demux1/4 -> Add1/4
  Add/1 -> Mux3/2
  Add1/1 -> Mux3/1
  Constant/1 -> Mux3/3

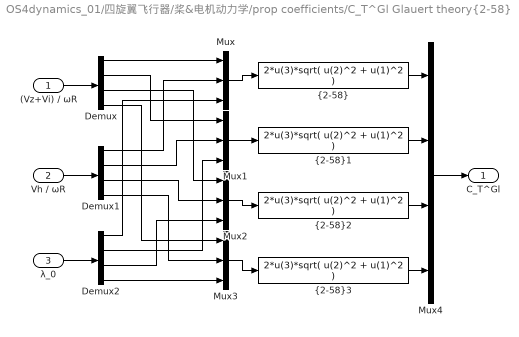
== system OS4dynamics_01/四旋翼飞行器/桨&电机动力学/prop coefficients/C_T^Gl Glauert theory{2-58} ==
  (Vz+Vi) / ωR : Inport
  Vh / ωR : Inport  Port=2
  λ_0 : Inport  Port=3
  Demux : Demux
  Demux1 : Demux
  Demux2 : Demux
  Mux{,1..3} (4 alike) : Mux  Inputs=3
  Mux4 : Mux
  {2-58}{,1..3} (4 alike) : Fcn  Expr=2*u(3)*sqrt( u(2)^2 + u(1)^2 )
  C_T^Gl : Outport
  wires:
  (Vz+Vi) / ωR/1 -> Demux/1
  λ_0/1 -> Demux2/1
  Vh / ωR/1 -> Demux1/1
  Demux2/4 -> Mux3/3
  Demux1/4 -> Mux3/2
  Demux/4 -> Mux3/1
  Demux/1 -> Mux/1
  Demux1/1 -> Mux/2
  Demux2/1 -> Mux/3
  Demux2/3 -> Mux2/3
  Demux1/3 -> Mux2/2
  Demux/3 -> Mux2/1
  Demux2/2 -> Mux1/3
  Demux1/2 -> Mux1/2
  Demux/2 -> Mux1/1
  Mux/1 -> "{2-58}"/1
  Mux1/1 -> "{2-58}1"/1
  Mux2/1 -> "{2-58}2"/1
  Mux3/1 -> "{2-58}3"/1
  "{2-58}"/1 -> Mux4/1
  "{2-58}1"/1 -> Mux4/2
  "{2-58}2"/1 -> Mux4/3
  "{2-58}3"/1 -> Mux4/4
  Mux4/1 -> C_T^Gl/1

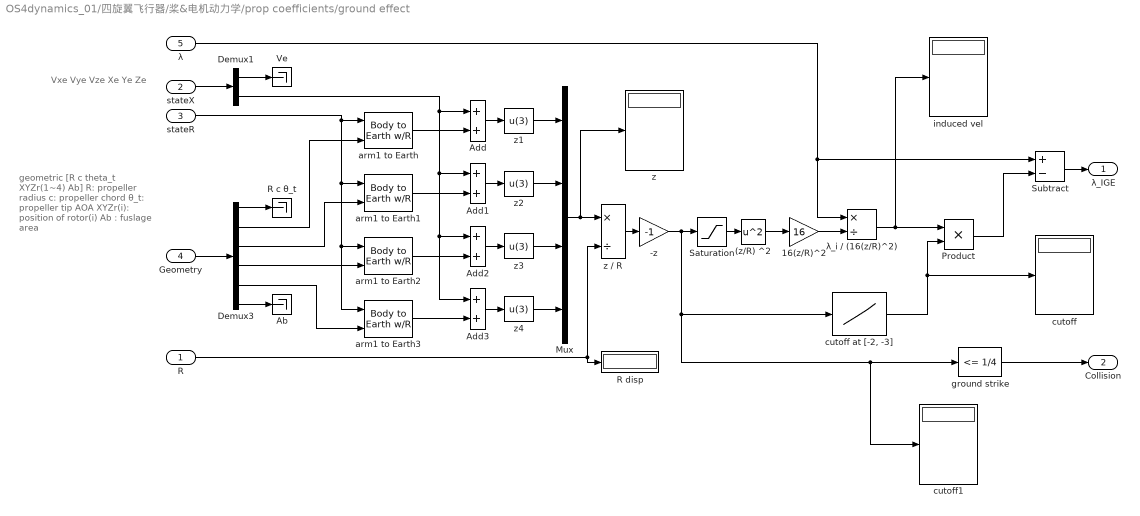
== system OS4dynamics_01/四旋翼飞行器/桨&电机动力学/prop coefficients/ground effect ==
  note: geometric
      | [R c theta_t XYZr(1~4) Ab]
      |
      | R: propeller radius
      | c: propeller chord
      | θ_t: propeller tip AOA
      | XYZr(i): position of rotor(i)
      | Ab : fuslage area
  note: Vxe Vye Vze
      |  Xe Ye Ze
  R : Inport
  stateX : Inport  Port=2
  stateR : Inport  Port=3
  Geometry : Inport  Port=4
  λ : Inport  Port=5
  (z/R) ^2 : Math  Operator=square  SaturateOnIntegerOverflow=on
  -z : Gain  Gain=-1
  16(z/R)^2 : Gain  Gain=16
  Ab : Terminator
  Add{,1..3} (4 alike) : Sum
  Demux1 : Demux  Outputs=[3 3]
  Demux3 : Demux  Outputs=[3 3 3 3 3 1]
  Mux : Mux
  Product : Product
  R c θ_t : Terminator
  R disp : Display
  Saturation : Saturate  UpperLimit=inf  LowerLimit=1/4
  Subtract : Sum  Inputs=+-
  Ve : Terminator
  arm1 to Earth{,1..3} (4 alike) : QuaternionLib/Body to Earth w//R
  cutoff : Display
  "cutoff at [-2, -3]" : Lookup_n-D  NumberOfTableDimensions=1  BreakpointsForDimension1=[2 3]  IndexSearchMethod=Linear search  Table="[1  0]"  ExtrapMethod=Clip  UseLastTableValue=on  InternalRulePriority=Speed  RndMeth=Simplest  InputSameDT=on
  cutoff1 : Display
  ground strike : simulink/Logic and Bit Operations/Compare To Constant  relop=<=  const=1/4  OutDataTypeStr=boolean
  induced vel : Display
  z : Display
  z / R : Product  Inputs=*/
  z{1..4} (4 alike) : Fcn  Expr=u(3)
  λ_i / (16(z/R)^2) : Product  Inputs=*/
  λ_IGE : Outport
  Collision : Outport  Port=2
  wires:
  stateX/1 -> Demux1/1
  Demux1/1 -> Ve/1
  stateR/1 -> arm1 to Earth3/1, arm1 to Earth2/1, arm1 to Earth1/1, arm1 to Earth/1
  Geometry/1 -> Demux3/1
  Demux3/1 -> R c θ_t/1
  Demux3/6 -> Ab/1
  Demux3/2 -> arm1 to Earth/2
  arm1 to Earth/1 -> Add/2
  Demux3/4 -> arm1 to Earth2/2
  Demux3/5 -> arm1 to Earth3/2
  Demux3/3 -> arm1 to Earth1/2
  Add/1 -> z1/1
  Add3/1 -> z4/1
  Add2/1 -> z3/1
  Add1/1 -> z2/1
  Demux1/2 -> Add3/1, Add2/1, Add1/1, Add/1
  arm1 to Earth1/1 -> Add1/2
  arm1 to Earth2/1 -> Add2/2
  arm1 to Earth3/1 -> Add3/2
  z2/1 -> Mux/2
  z3/1 -> Mux/3
  z4/1 -> Mux/4
  z1/1 -> Mux/1
  Mux/1 -> z/1, z / R/1
  (z/R) ^2/1 -> 16(z/R)^2/1
  Saturation/1 -> (z/R) ^2/1
  R/1 -> z / R/2, R disp/1
  λ/1 -> λ_i / (16(z/R)^2)/1, Subtract/1
  16(z/R)^2/1 -> λ_i / (16(z/R)^2)/2
  λ_i / (16(z/R)^2)/1 -> induced vel/1, Product/1
  "cutoff at [-2, -3]"/1 -> cutoff/1, Product/2
  Subtract/1 -> λ_IGE/1
  Product/1 -> Subtract/2
  z / R/1 -> -z/1
  ground strike/1 -> Collision/1
  -z/1 -> cutoff1/1, ground strike/1, "cutoff at [-2, -3]"/1, Saturation/1

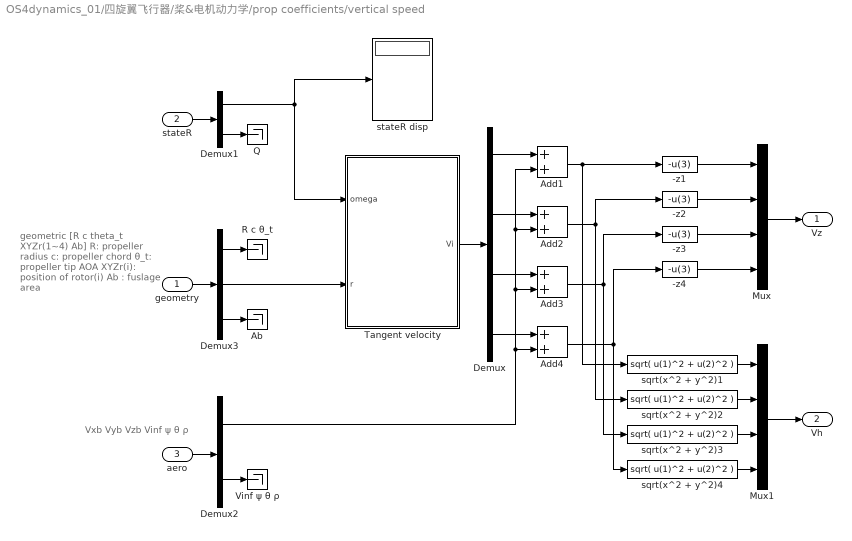
== system OS4dynamics_01/四旋翼飞行器/桨&电机动力学/prop coefficients/vertical speed ==
  note: Vxb Vyb Vzb
      | Vinf ψ θ ρ
  note: geometric
      | [R c theta_t XYZr(1~4) Ab]
      |
      | R: propeller radius
      | c: propeller chord
      | θ_t: propeller tip AOA
      | XYZr(i): position of rotor(i)
      | Ab : fuslage area
  geometry : Inport
  stateR : Inport  Port=2
  aero : Inport  Port=3
  -z{1..4} (4 alike) : Fcn  Expr=-u(3)
  Ab : Terminator
  Add{1..4} (4 alike) : Sum
  Demux : Demux  Outputs=[3 3 3 3]
  Demux1 : Demux  Outputs=[3 4]
  Demux2 : Demux  Outputs=[3 4]
  Demux3 : Demux  Outputs=[3 12 1]
  Mux : Mux
  Mux1 : Mux
  Q : Terminator
  R c θ_t : Terminator
  Tangent velocity : MATLAB Function  TreatAsAtomicUnit=on
  Vinf ψ θ ρ : Terminator
  sqrt(x^2 + y^2){1..4} (4 alike) : Fcn  Expr=sqrt( u(1)^2 + u(2)^2 )
  stateR disp : Display
  Vz : Outport
  Vh : Outport  Port=2
  wires:
  geometry/1 -> Demux3/1
  stateR/1 -> Demux1/1
  Demux1/1 -> Tangent velocity/1(omega), stateR disp/1
  Demux3/2 -> Tangent velocity/2(r)
  Demux3/1 -> R c θ_t/1
  Demux3/3 -> Ab/1
  Demux1/2 -> Q/1
  aero/1 -> Demux2/1
  Demux2/2 -> Vinf ψ θ ρ/1
  Tangent velocity/1(Vi) -> Demux/1
  Demux/1 -> Add1/1
  Demux/2 -> Add2/1
  Demux/3 -> Add3/1
  Demux/4 -> Add4/1
  Demux2/1 -> Add4/2, Add3/2, Add1/2, Add2/2
  Add1/1 -> sqrt(x^2 + y^2)1/1, -z1/1
  Add2/1 -> -z2/1, sqrt(x^2 + y^2)2/1
  Add3/1 -> -z3/1, sqrt(x^2 + y^2)3/1
  Add4/1 -> -z4/1, sqrt(x^2 + y^2)4/1
  -z1/1 -> Mux/1
  Mux/1 -> Vz/1
  -z2/1 -> Mux/2
  -z3/1 -> Mux/3
  -z4/1 -> Mux/4
  sqrt(x^2 + y^2)2/1 -> Mux1/2
  sqrt(x^2 + y^2)4/1 -> Mux1/4
  sqrt(x^2 + y^2)1/1 -> Mux1/1
  sqrt(x^2 + y^2)3/1 -> Mux1/3
  Mux1/1 -> Vh/1

== matlab function OS4dynamics_01/四旋翼飞行器/桨&电机动力学/R cross F ==
  data: Thrust input; M_hr output; geo input
function M_hr = RxF(Thrust, geo)
M_hr = zeros(3,1);
for i = 1:4
    M_hr = M_hr + cross(geo(i*3+1:i*3+3),[0; 0; -Thrust(i)]);
end
end

== matlab function OS4dynamics_01/四旋翼飞行器/桨&电机动力学/prop coefficients/vertical speed/Tangent velocity ==
  data: omega input; Vi output; r input
function Vi = OmegaCrossR4(omega,r)
Vi = zeros(1,12);
for i = 1:4
    Vi(i*3-2:i*3) = cross(omega,r(i*3-2:i*3));
end
end
